simulink model "fig2_18_simulink"  (R2021b)
settings: Solver=ode45  StartTime=0.0  StopTime=30  RelTol=1e-3  EnableMultiTasking=on
model workspace (MAT data in the model file):
  X0 = 0
values from neighbouring files (symbols this model uses):
  B = 2.1    [fig2_19.m]
settings Model: Creator=One Informatic  LastModifiedBy=One Informatic
settings DataIOCC: LimitDataPoints=on  SaveFormat=Array  SignalLoggingSaveFormat=ModelDataLogs  ReturnWorkspaceOutputs=off  SignalLoggingName=sigsOut
settings DebuggingCC: SaveWithParameterizedLinksMsg=none  UnderspecifiedInitializationDetection=Classic  MergeDetectMultiDrivingBlocksExec=none  SignalResolutionControl=TryResolveAllWithWarning  MultiTaskDSMMsg=warning  MultiTaskCondExecSysMsg=none
settings HardwareCC: ProdBitPerPointer=32  ProdBitPerSizeT=32  ProdBitPerPtrDiffT=32  ProdLargestAtomicFloat=None  ProdIntDivRoundTo=Undefined  ProdEndianess=Unspecified  ProdWordSize=32  ProdHWDeviceType=32-bit Generic  TargetUnknown=on
settings ModelReferenceCC: PropagateSignalLabelsOutOfModel=off
settings GRTTargetCC: CombineOutputUpdateFcns=off  GRTInterface=on
settings ConfigComp: CovMetricSettings=dw  CovSaveCumulativeToWorkspaceVar=on  CovSaveSingleToWorkspaceVar=on

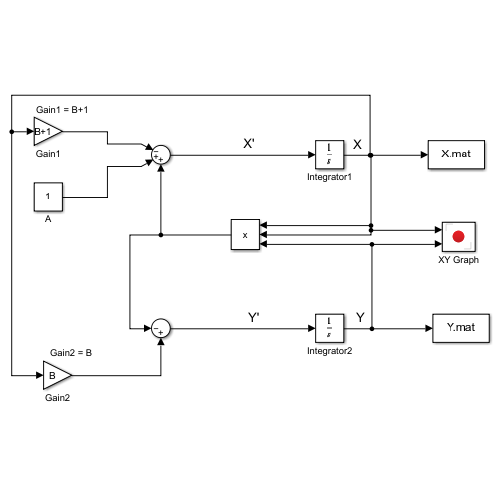
[thumbnail: Simulink's stored preview of the top-level diagram]
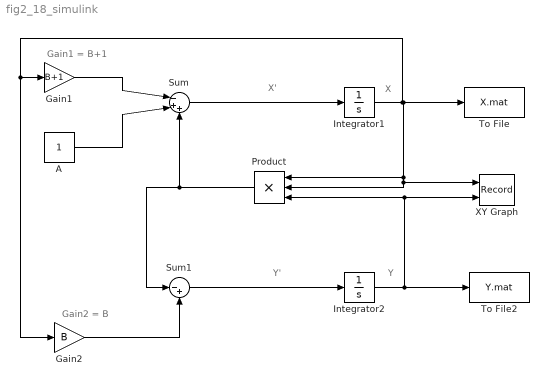
== system fig2_18_simulink ==
  note: Gain1 = B+1
  note: X'
  note: X
  note: Y'
  note: Y
  note: Gain2 = B
  A : Constant
  Gain1 : Gain  Gain=B+1
  Gain2 : Gain  Gain=B
  Integrator1 : Integrator  InitialCondition=2
  Integrator2 : Integrator  InitialCondition=3
  Product : Product  Inputs=3
  Sum : Sum  Inputs=|-++
  Sum1 : Sum  Inputs=|-+
  To File : ToFile  Filename=X.mat  MatrixName=X  SampleTime=0.001
  To File2 : ToFile  Filename=Y.mat  MatrixName=Y  SampleTime=0.001
  XY Graph : Record  FileSettingsInternal="{\"entries\":[{\"content\":{\"excelSettings\":{\"content\":{},\"type\":\"Streamout.ExcelSettings\"}},\"type\":\"Streamout.FileSettingStorage\",\"uuid\":\"c2565e3c-df81-4bf1-9553-0a324edf4095\"}],\"packageUris\":[\"http://schema.mathworks.com/mf0/streamout_blocks/R2020a\"],\"version\":\"1.0\"}"  Layout=[1 1]  SignalsInternal="{\"entries\":[{\"content\":{\"signals\":[{\"content\":{\"blockPath\":[\"fig2_18_simulink/XY Graph\"],\"channel\":[],\"dimensions\":[1],\"domain\":\"fig2_18_simulink/XY Graph\",\"lineColor\":\"#a2142f\",\"plots\":[],\"port\":1,\"sid\":[\"\"],\"signalID\":1080,\"signalName\":\"Integrator1\"},\"type\":\"RecordBlkView.Signal\",\"uuid\":\"8f16423f-890a-4f7d-94a4-8240eb80c208\"},{\"content\":{\"blockPath\":[\"fig2_18_simulink/XY Graph\"],\"channel\":[],\"dimensions\":[1],\"domain\":\"fig2_18_simulink/XY Graph\",\"lineColor\":\"#139fff\",\"plots\":[],\"port\":2,\"sid\":[\"\"],\"signalID\":1084,\"signalName\":\"Integrator2\"},\"type\":\"RecordBlkView.Signal\",\"uuid\":\"87acebde-3a10-401b-b877-32bc43222dd8\"}]},\"type\":\"RecordBlkView.InputSignals\",\"uuid\":\"ecc116d0-87f7-470e-b1a0-b98cd6b82b24\"}],\"packageUris\":[\"http://schema.mathworks.com/mf0/streamout_blocks/R2020a\"],\"version\":\"1.0\"}"  VisualizationBindings="{\"xyplotplugin\":{\"info\":[{\"series\":[],\"subplotID\":1}]}}"  CompatibilityTag=XY
  wires:
  A/1 -> Sum/2
  Gain1/1 -> Sum/1
  Product/1 -> Sum/3, Sum1/1
  Sum1/1 -> Integrator2/1
  Gain2/1 -> Sum1/2
  Sum/1 -> Integrator1/1
  Integrator1/1 -> Gain2/1, Gain1/1, Product/2, XY Graph/1, Product/1, To File/1
  Integrator2/1 -> To File2/1, XY Graph/2, Product/3
